simulink model "Tuner"  (R2013b)
settings: Solver=ode4  StartTime=0.0  StopTime=70  FixedStep=0.01  RelTol=1e-3
undefined symbols (not defined in the file or in its folder): G6
libraries: cstblocks x1, simulink x1
settings Model: Creator=stelmo  LastModifiedBy=stelmo

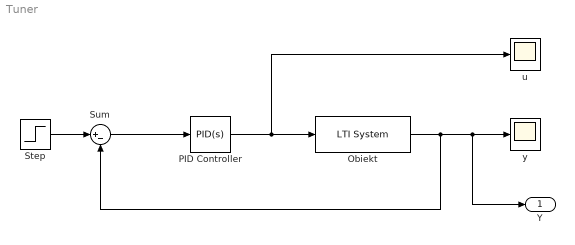
== system Tuner ==
  Obiekt : cstblocks/LTI System  sys=G6(8)  IC=[]
  PID Controller : simulink/Continuous/PID Controller  Controller=PID  TimeDomain=Continuous-time  SampleTime=1  IntegratorMethod=Forward Euler  FilterMethod=Forward Euler  Form=Parallel  P=0.660160714279233  I=0.00384405342086614  D=0.151151374725753  N=76.1520644057718  InitialConditionSource=internal  InitialConditionForIntegrator=0  InitialConditionForFilter=0  ExternalReset=none  LimitOutput=off  UpperSaturationLimit=inf  LowerSaturationLimit=-inf  LinearizeAsGain=on  AntiWindupMode=none  Kb=1  TrackingMode=off  Kt=1  PParamMin=[]  PParamMax=[]  IParamMin=[]  IParamMax=[]  DParamMin=[]  DParamMax=[]  NParamMin=[]  NParamMax=[]  KbParamMin=[]  KbParamMax=[]  KtParamMin=[]  KtParamMax=[]  POutMin=[]  POutMax=[]  IOutMin=[]  IOutMax=[]  DOutMin=[]  DOutMax=[]  NOutMin=[]  NOutMax=[]  KbOutMin=[]  KbOutMax=[]  KtOutMin=[]  KtOutMax=[]  IntegratorOutMin=[]  IntegratorOutMax=[]  FilterOutMin=[]  FilterOutMax=[]  SumOutMin=[]  SumOutMax=[]  SumI1OutMin=[]  SumI1OutMax=[]  SumI2OutMin=[]  SumI2OutMax=[]  SumI3OutMin=[]  SumI3OutMax=[]  SumDOutMin=[]  SumDOutMax=[]  SaturationOutMin=[]  SaturationOutMax=[]  IntegratorContinuousStateAttributes=''  IntegratorStateMustResolveToSignalObject=off  IntegratorRTWStateStorageClass=Auto  FilterContinuousStateAttributes=''  FilterStateMustResolveToSignalObject=off  FilterRTWStateStorageClass=Auto
  Step : Step  SampleTime=0
  Sum : Sum  Inputs=|+-
  u : Scope
  y : Scope
      settings: MaxDataPoints=50000000
  Y : Outport
  wires:
  Step/1 -> Sum/1
  Obiekt/1 -> Y/1, y/1, Sum/2
  PID Controller/1 -> Obiekt/1, u/1
  Sum/1 -> PID Controller/1
